simulink model "BRS_Tay"  (R2015b)
settings: Solver=FixedStepDiscrete  StartTime=0.0  StopTime=1.0  FixedStep=1.0  RelTol=1e-3
libraries: taXlibrary x14
settings Model: Creator=emmert  LastModifiedBy=thomas
settings DataIOCC: SaveFormat=Array  SignalLoggingSaveFormat=ModelDataLogs
settings OptimizationCC: ExpressionDepthLimit=2147483647
settings DebuggingCC: UnderspecifiedInitializationDetection=Classic  MergeDetectMultiDrivingBlocksExec=none  SolverPrmCheckMsg=warning  FcnCallInpInsideContextMsg=EnableAllAsWarning  StateNameClashWarn=warning
settings HardwareCC: ProdBitPerPointer=32  ProdLargestAtomicFloat=None  ProdIntDivRoundTo=Undefined  ProdEndianess=Unspecified  ProdWordSize=32  ProdHWDeviceType=32-bit Generic
settings GRTTargetCC: GeneratePreprocessorConditionals=Disable all  CombineOutputUpdateFcns=off  GRTInterface=on
settings ConfigComp: CovModelRefEnable=Off  CovSFcnEnable=off

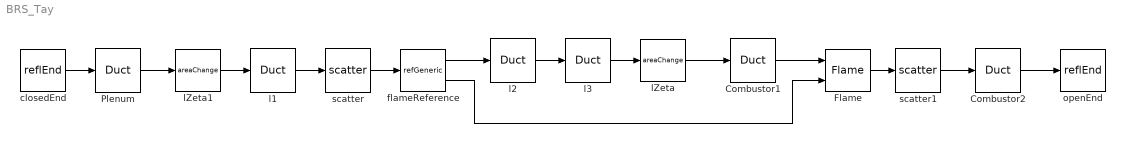
== system BRS_Tay ==
  Combustor1 : taXlibrary/Duct  element=Duct  order=3  minres=20  l=0.00403  sensorPositions=[]
      settings: AttributesFormatString=%<l> m
  Combustor2 : taXlibrary/Duct  element=Duct  order=3  minres=20  l=0.7-0.00403  sensorPositions=[]
      settings: AttributesFormatString=%<l> m
  Flame : taXlibrary/Flame  element=rankineHugoniot  nRef=1  Mach=0.001056*101325/(287.04*293)*11.3/(101325/(287.04*1930)*0.0081*sqrt(1.4*287.04*1930))  rho=101325/(287.04*1930)  c=sqrt(1.4*287.04*1930)
  Plenum : taXlibrary/Duct  element=Duct  order=3  minres=20  l=0.17  sensorPositions=[]
      settings: AttributesFormatString=%<l> m
  closedEnd : taXlibrary/reflEnd  element=reflEnd  loc=Upstream  r=1  A=0.031416  Mach=11.3*0.001056/0.031416/sqrt(1.4*287.04*293)  rho=101325/(287.04*293)  c=sqrt(1.4*287.04*293)
      settings: AttributesFormatString=%<r>
  flameReference : taXlibrary/refGeneric  element=reference  filename=Testcases/model_Luis_30kW_9.5%.mat  modelname=model  active=on
      settings: AttributesFormatString=%<modelname>
  l1 : taXlibrary/Duct  element=Duct  order=3  minres=20  l=0.11  sensorPositions=[]
      settings: AttributesFormatString=%<l> m
  l2 : taXlibrary/Duct  element=Duct  order=3  minres=20  l=0.025  sensorPositions=[]
      settings: AttributesFormatString=%<l> m
  l3 : taXlibrary/Duct  element=Duct  order=3  minres=20  l=0.045  sensorPositions=[]
      settings: AttributesFormatString=%<l> m
  lZeta : taXlibrary/areaChange  element=lZeta  zeta=0  lred=0  leff=0  l=1  A=90*90/1000^2
  lZeta1 : taXlibrary/areaChange  element=lZeta  zeta=0  lred=0  leff=0  l=1  A=pi/4*((40/1000)^2-(16/1000)^2)
  openEnd : taXlibrary/reflEnd  element=reflEnd  loc=Downstream  r=-1  A=[]  Mach=[]  rho=[]  c=[]
      settings: AttributesFormatString=%<r>
  scatter : taXlibrary/scatter  element=scatteringDummy  loc=Upstream
  scatter1 : taXlibrary/scatter  element=scatteringDummy  loc=Downstream
  wires:
  Combustor1/1 -> Flame/1
  Flame/1 -> scatter1/1
  l3/1 -> lZeta/1
  lZeta/1 -> Combustor1/1
  flameReference/1 -> l2/1
  flameReference/2 -> Flame/2
  scatter/1 -> flameReference/1
  lZeta1/1 -> l1/1
  Plenum/1 -> lZeta1/1
  l1/1 -> scatter/1
  scatter1/1 -> Combustor2/1
  closedEnd/1 -> Plenum/1
  l2/1 -> l3/1
  Combustor2/1 -> openEnd/1
